simulink model "codingexample_Hamming"  (R2023a)
settings: Solver=VariableStepAuto  StartTime=0.0  StopTime=inf  RelTol=1e-3
values from neighbouring files (symbols this model uses):
  msglength = 4    [codingexample_control.m]
libraries: commdigbbndpm3 x4, commchan3 x2, commsink2 x2, commblkcod2 x2, commrandsrc3 x1
settings Model: SimulationMode=accelerator  Creator=Vili  LastModifiedBy=arttu
settings DataIOCC: SaveOutput=off  SignalLogging=off  DSMLogging=off  SaveTime=off  ReturnWorkspaceOutputs=off
settings DebuggingCC: UnconnectedInputMsg=warning  UnconnectedOutputMsg=warning  UnconnectedLineMsg=warning
settings ModelReferenceCC: EnableRefExpFcnMdlSchedulingChecks=on
settings RTWCC: DLArmComputeVersion=19.05

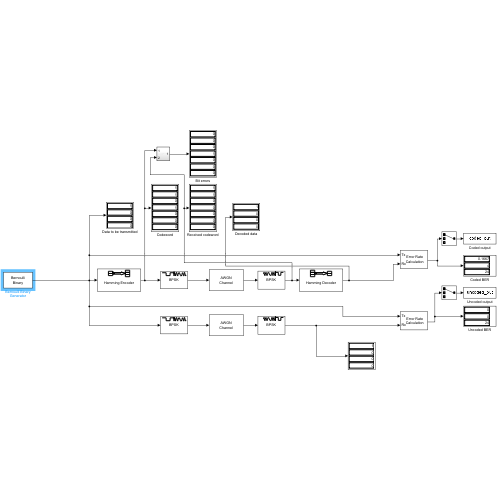
[thumbnail: Simulink's stored preview of the top-level diagram]
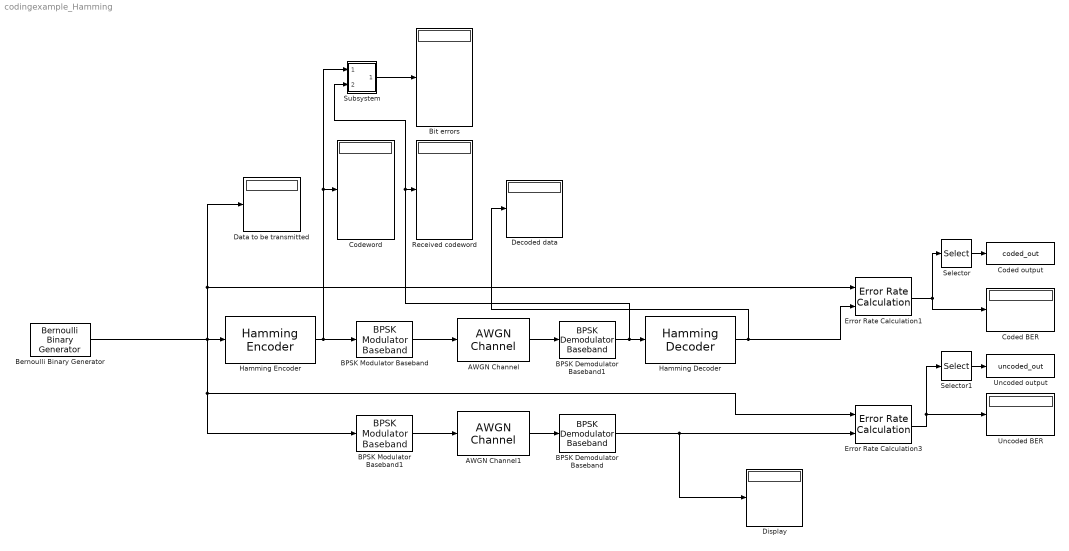
== system codingexample_Hamming ==
  AWGN Channel : commchan3/AWGN Channel  LegacyMode=on  NoiseMethod="Signal to noise ratio  (SNR)"  noiseMode="Signal to noise ratio  (Eb/No)"  EbNo=EbN0  EsNo=10  SNR=10  BitsPerSymbol=1  SignalPower=1  SamplesPerSymbol=1  SymbolPeriod=1  VarianceSource=Parameter  Variance=1  RandomStream=Global stream  Seed=963  SimulateUsing=Code generation
  AWGN Channel1 : commchan3/AWGN Channel  LegacyMode=on  NoiseMethod="Signal to noise ratio  (SNR)"  noiseMode="Signal to noise ratio  (Eb/No)"  EbNo=EbN0  EsNo=10  SNR=10  BitsPerSymbol=1  SignalPower=1  SamplesPerSymbol=1  SymbolPeriod=1  VarianceSource=Parameter  Variance=1  RandomStream=Global stream  Seed=963  SimulateUsing=Code generation
  BPSK Demodulator Baseband : commdigbbndpm3/BPSK Demodulator Baseband  DecType=Hard decision  VarSource=Dialog  Variance=1  Ph=0  outDtype=Inherit via internal rule  derotateFactorWordLen=16  derotateFactorDataTypeStr=Inherit: Same word length as input  derotateFactorLastDataTypeStr=Inherit: Same word length as input
  BPSK Demodulator Baseband1 : commdigbbndpm3/BPSK Demodulator Baseband  DecType=Hard decision  VarSource=Dialog  Variance=1  Ph=0  outDtype=Inherit via internal rule  derotateFactorWordLen=16  derotateFactorDataTypeStr=Inherit: Same word length as input  derotateFactorLastDataTypeStr=Inherit: Same word length as input
  BPSK Modulator Baseband : commdigbbndpm3/BPSK Modulator Baseband  Ph=0  outDtype=double  outWordLen=16  outUDDataType=sfix(16)  outFracLenMode=Best precision  outFracLen=15  outDataTypeStr=double  outLastDataTypeStr=double
  BPSK Modulator Baseband1 : commdigbbndpm3/BPSK Modulator Baseband  Ph=0  outDtype=double  outWordLen=16  outUDDataType=sfix(16)  outFracLenMode=Best precision  outFracLen=15  outDataTypeStr=double  outLastDataTypeStr=double
  Bernoulli Binary Generator : commrandsrc3/Bernoulli Binary Generator  ProbabilityOfZero=0.5  SeedSource=Parameter  Seed=1155  SampleTime=1  SamplesPerFrame=msglength  OutputDataType=double  SimulateUsing=Interpreted execution
  Bit errors : Display
  Coded BER : Display
  Coded output : ToWorkspace  VariableName=coded_out  SaveFormat=Timeseries  SampleTime=-1
  Codeword : Display
  Data to be transmitted : Display
  Decoded data : Display
  Display : Display
  Error Rate Calculation1 : commsink2/Error Rate Calculation  N=0  st_delay=0  cp_mode=Entire frame  subframe=[]  PMode=Port  WsName=ErrorVec  RsMode2=off  stop=on  numErr=1000  maxBits=1e6
  Error Rate Calculation3 : commsink2/Error Rate Calculation  N=0  st_delay=0  cp_mode=Entire frame  subframe=[]  PMode=Port  WsName=ErrorVec  RsMode2=off  stop=on  numErr=1000  maxBits=1e6
  Hamming Decoder : commblkcod2/Hamming Decoder  n=cdlength  k=msglength
  Hamming Encoder : commblkcod2/Hamming Encoder  n=cdlength  k=msglength
  Received codeword : Display
  Selector : Selector  InputPortWidth=3  IndexOptions=Index vector (dialog)  Indices=1  OutputSizes=1
  Selector1 : Selector  InputPortWidth=3  IndexOptions=Index vector (dialog)  Indices=1  OutputSizes=1
  Subsystem : Subsystem
  Uncoded BER : Display
  Uncoded output : ToWorkspace  VariableName=uncoded_out  SaveFormat=Timeseries  SampleTime=-1
  wires:
  BPSK Demodulator Baseband1/1 -> Subsystem/2(Input), Received codeword/1, Hamming Decoder/1
  Hamming Encoder/1 -> BPSK Modulator Baseband/1, Subsystem/1(In1), Codeword/1
  Bernoulli Binary Generator/1 -> Hamming Encoder/1, Error Rate Calculation1/1, Data to be transmitted/1, Error Rate Calculation3/1, BPSK Modulator Baseband1/1
  Hamming Decoder/1 -> Error Rate Calculation1/2, Decoded data/1
  Error Rate Calculation1/1 -> Selector/1, Coded BER/1
  BPSK Demodulator Baseband/1 -> Display/1, Error Rate Calculation3/2
  Error Rate Calculation3/1 -> Selector1/1, Uncoded BER/1
  Subsystem/1(Out1) -> Bit errors/1
  BPSK Modulator Baseband/1 -> AWGN Channel/1
  AWGN Channel/1 -> BPSK Demodulator Baseband1/1
  BPSK Modulator Baseband1/1 -> AWGN Channel1/1
  AWGN Channel1/1 -> BPSK Demodulator Baseband/1
  Selector1/1 -> Uncoded output/1
  Selector/1 -> Coded output/1

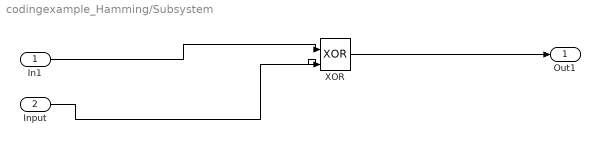
== system codingexample_Hamming/Subsystem ==
  In1 : Inport
  Input : Inport  Port=2
  XOR : Logic  Operator=XOR  IconShape=distinctive  AllPortsSameDT=off  OutDataTypeStr=boolean
  Out1 : Outport
  wires:
  In1/1 -> XOR/1
  Input/1 -> XOR/2
  XOR/1 -> Out1/1
